simulink model "SigNetLabExp3code_19CS30031"  (R2020a)
settings: Solver=ode23t  StartTime=0.0  StopTime=10  RelTol=1e-3
libraries: powerlib x9, powerlib_meascontrol x2
settings Model: Creator=nisar  LastModifiedBy=nisar

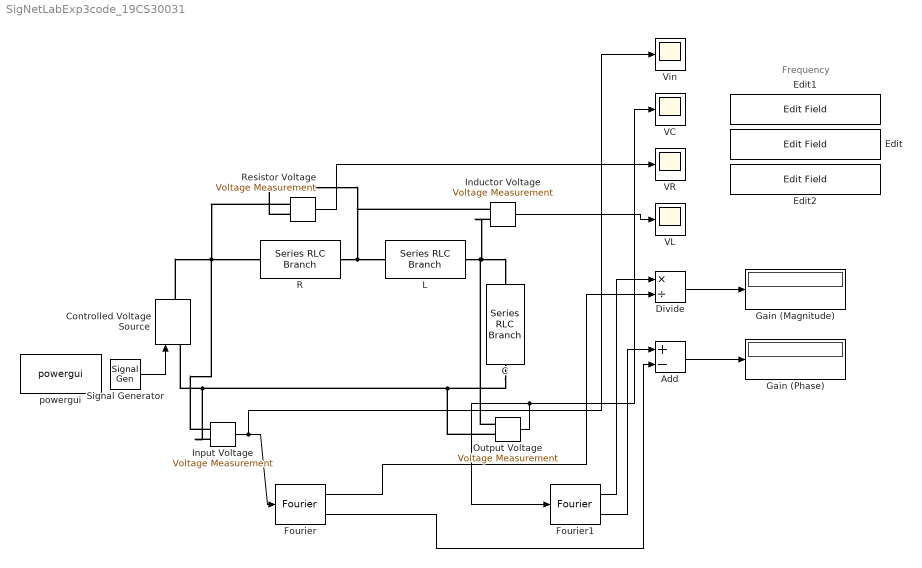
== system SigNetLabExp3code_19CS30031 ==
  note: Frequency
  Add : Sum  Inputs=+-
  C : powerlib/Elements/Series RLC Branch  LConnTagsString=__new0  RConnTagsString=__new0  BranchType=C  Resistance=1  Inductance=1e-3  SetiL0=off  InitialCurrent=0  Capacitance=1e-7  Setx0=off  InitialVoltage=0  Measurements=None
  Controlled Voltage Source : powerlib/Electrical Sources/Controlled Voltage Source  Initialize=on  Source_Type=AC  Amplitude=0  Phase=0  Frequency=0  Measurements=None
  Divide : Product  Inputs=*/
  Edit : EditField  LabelPosition=Hide  ShowInitialText=on  Alignment=Center
  Edit1 : EditField  LabelPosition=Hide  ShowInitialText=on  Alignment=Center
  Edit2 : EditField  LabelPosition=Hide  ShowInitialText=on  Alignment=Center
  Fourier : powerlib_meascontrol/Measurements/Fourier  Freq=300  n=1  InInit=[0, 0]  Ts=0
  Fourier1 : powerlib_meascontrol/Measurements/Fourier  Freq=300  n=1  InInit=[0, 0]  Ts=0
  Gain (Magnitude) : Display
  Gain (Phase) : Display
  Inductor Voltage : powerlib/Measurements/Voltage Measurement  PhasorSimulation=off  OutputType=Complex  PSBequivalent=0
  Input Voltage : powerlib/Measurements/Voltage Measurement  PhasorSimulation=off  OutputType=Complex  PSBequivalent=0
  L : powerlib/Elements/Series RLC Branch  LConnTagsString=__new0  RConnTagsString=__new0  BranchType=L  Resistance=1  Inductance=0.1  SetiL0=off  InitialCurrent=0  Capacitance=1e-6  Setx0=off  InitialVoltage=0  Measurements=None
  Output Voltage : powerlib/Measurements/Voltage Measurement  PhasorSimulation=off  OutputType=Complex  PSBequivalent=0
  R : powerlib/Elements/Series RLC Branch  LConnTagsString=__new0  RConnTagsString=__new0  BranchType=R  Resistance=400  Inductance=0  SetiL0=off  InitialCurrent=0  Capacitance=1e-6  Setx0=off  InitialVoltage=0  Measurements=None
  Resistor Voltage : powerlib/Measurements/Voltage Measurement  PhasorSimulation=off  OutputType=Complex  PSBequivalent=0
  Signal Generator : SignalGenerator  Amplitude=5  Frequency=300
  VC : Scope
  VL : Scope
  VR : Scope
  Vin : Scope
  powergui : powerlib/powergui  Priority=1  SimulationMode=Continuous  SampleTime=50e-6  frequency=60  Iterations=50  frequencyindice=0  Pbase=100e6  ErrMax=1e-4  UnitsV=kV  UnitsW=MW  buscounter=0  FunctionMessages=off  echomessages=off  EnableUseOfTLC=off  CurrentSourceSwitches=off  DisableSnubberDevices=off  DisableRonSwitches=off  DisableVfSwitches=off  DisplayEquations=off  AutomaticDiscreteSolvers=off  SolverType=Tustin/Backward Euler (TBE)  Interpol=off  ExternalGateDelay=off  methode=off  Ts=100  x0status=blocks  SPID=on  SwTol=0  HookPort=off  NonlinearTolerance=1e-4  nMaxIteration=100  ContinueOnMaxIteration=off  RestoreLinks=warning  ResistiveCurrentMeasurement=off  Frange=[0:2:500]  Ylog=off  Xlog=on  ShowGrid=off  save=off  variable=ZData  structure=0  ZoomFFT=off  StartTime=0.0  cycles=1  DisplayStyle=1  fundamental=60  FreqAxis=off  MaxFrequency=1000  frequencyindicesteady=1  RmsSteady=1  display=off
  wires:
  Signal Generator/1 -> Controlled Voltage Source/1
  Input Voltage/1 -> Vin/1, Fourier/1
  Fourier1/1 -> Divide/1
  Fourier/1 -> Divide/2
  Fourier1/2 -> Add/1
  Fourier/2 -> Add/2
  Divide/1 -> Gain (Magnitude)/1
  Add/1 -> Gain (Phase)/1
  Output Voltage/1 -> VC/1, Fourier1/1
  Inductor Voltage/1 -> VL/1
  Resistor Voltage/1 -> VR/1
  connections:
  Controlled Voltage Source/RConn1 -- Resistor Voltage/LConn1 -- Input Voltage/LConn1 -- R/LConn1
  R/RConn1 -- Inductor Voltage/LConn1 -- Resistor Voltage/LConn2 -- L/LConn1
  L/RConn1 -- Inductor Voltage/LConn2 -- C/LConn1 -- Output Voltage/LConn1
  C/RConn1 -- Output Voltage/LConn2 -- Input Voltage/LConn2 -- Controlled Voltage Source/LConn1
